simulink library "hal"  (Simulink 8.2)
settings: Solver=ode45  SolverMode=SingleTasking  StartTime=0.0  StopTime=10.0  RelTol=1e-3
PostLoadFcn:
  | , if any(exist('dsrtsu_mdlpostloadfcn', 'file') == [2, 3, 6]), try dsrtsu_mdlpostloadfcn('Execute', bdroot); catch fprintf('Error in PostLoadFcn (dsrtsu_mdlpostloadfcn) for model "%s":\n %s\n', bdroot, lasterr); end, end,
values from neighbouring files (symbols this model uses):
  INVALID_ABS1_TIMEOUT = single(0.03)    [hal_def.m]
  INVALID_ABS2_TIMEOUT = single(0.03)    [hal_def.m]
  INVALID_ABS3_TIMEOUT = single(0.03)    [hal_def.m]
  INVALID_ABS4_TIMEOUT = single(0.03)    [hal_def.m]
  INVALID_AC1_TIMEOUT = single(0.3)    [hal_def.m]
  INVALID_BCM1_TIMEOUT = single(0.6)    [hal_def.m]
  INVALID_BCM2_TIMEOUT = single(0.06)    [hal_def.m]
  INVALID_BOOSTER_VAC = uint32(255)    [hal_def.m]
  INVALID_CUR_VEHDECE = uint32(255)    [hal_def.m]
  INVALID_CURBRAKEDECE_REQ = uint32(255)    [hal_def.m]
  INVALID_CURSTEERANG_REQ = uint32(65535)    [hal_def.m]
  INVALID_CURSTEERTQ_REQ = uint32(255)    [hal_def.m]
  INVALID_ECM1_TIMEOUT = single(0.03)    [hal_def.m]
  INVALID_ECM2_TIMEOUT = single(0.03)    [hal_def.m]
  INVALID_ECM3_TIMEOUT = single(0.03)    [hal_def.m]
  INVALID_ECM9_TIMEOUT = single(0.03)    [hal_def.m]
  INVALID_ENG_TORQUE_FRICTIONAL = uint32(255)    [hal_def.m]
  INVALID_ENG_TORQUE_INDICATED = uint32(255)    [hal_def.m]
  INVALID_ENG_TORQUE_INDICATEDCOR = uint32(255)    [hal_def.m]
  INVALID_ENG_TQ_MAX = uint32(65535)    [hal_def.m]
  INVALID_ENG_TQ_MIN = uint32(65535)    [hal_def.m]
  INVALID_EPAS2_TIMEOUT = single(0.03)    [hal_def.m]
  INVALID_EPAS3_TIMEOUT = single(0.03)    [hal_def.m]
  INVALID_EPB1_TIMEOUT = single(0.12)    [hal_def.m]
  INVALID_EPS_BATTVOLT = uint32(251)    [hal_def.m]
  INVALID_ESC_BATTVOLT = uint32(251)    [hal_def.m]
  INVALID_GRADE = uint32(255)    [hal_def.m]
  INVALID_HCU3_TIMEOUT = single(0.03)    [hal_def.m]
  INVALID_HCU4_TIMEOUT = single(0.03)    [hal_def.m]
  INVALID_HMI1_TIMEOUT = single(0.03)    [hal_def.m]
  INVALID_HMI2_TIMEOUT = single(0.03)    [hal_def.m]
  INVALID_LAT_ACC = uint32(255)    [hal_def.m]
  INVALID_LONG_ACC = uint32(255)    [hal_def.m]
  INVALID_MC_PRESSURE = uint32(2047)    [hal_def.m]
  INVALID_METER1_TIMEOUT = single(0.3)    [hal_def.m]
  INVALID_METER3_TIMEOUT = single(0.3)    [hal_def.m]
  INVALID_METER_VEHSPD = uint32(2048)    [hal_def.m]
  INVALID_ODO_METER = uint32(1000000)    [hal_def.m]
  INVALID_OUTSIDE_TEMP = uint32(96)    [hal_def.m]
  INVALID_PARKBRAKEBIND_STAT = uint32(3)    [hal_def.m]
  INVALID_SAS1_TIMEOUT = single(0.03)    [hal_def.m]
  INVALID_SAS_ANGLE = uint32(65535)    [hal_def.m]
  INVALID_SHIFTER_POSN = uint32(6)    [hal_def.m]
  INVALID_TCM1_TIMEOUT = single(0.03)    [hal_def.m]
  INVALID_TCM2_TIMEOUT = single(0.03)    [hal_def.m]
  INVALID_VCU1_TIMEOUT = single(0.03)    [hal_def.m]
  INVALID_VCU2_TIMEOUT = single(0.03)    [hal_def.m]
  INVALID_VEH_CRASH = uint32(15)    [hal_def.m]
  INVALID_VEH_SPD = uint32(2048)    [hal_def.m]
  INVALID_WHEEL_SPD = uint32(16377)    [hal_def.m]
  INVALID_YAW_RATE = uint32(2001)    [hal_def.m]
undefined symbols (not defined in the file or in its folder): C_TASK_5MS_S, FALSE, INVALID_CURPTTORQ_REQ, KHAL_MssgIdObj1_num, KHAL_MssgIdObj2_num, KHAL_MssgIdObjStatus_num, TRUE
libraries: simulink x92
(part 8 of 8)

== system hal/dHAL_IN/dHAL_IN_ABS/BO_864_ABS2_8_ABS/IcM ==
  LowByte : Inport
  HighByte : Inport  Port=2
  Bitwise Operator : simulink/Logic and Bit Operations/Bitwise Operator  logicop=OR  UseBitMask=off  NumInputPorts=2  BitMask=bin2dec('11011001')  BitMaskRealWorld=Stored Integer
  Cast1 : DataTypeConversion  OutDataTypeStr=uint16  RndMeth=Zero
  Cast45 : DataTypeConversion  OutDataTypeStr=uint16  RndMeth=Zero
  Shift Arithmetic : ArithShift  BitShiftNumber=-4
  Shift Arithmetic1 : ArithShift  BitShiftNumber=4
  HighLowByte : Outport
  wires:
  Shift Arithmetic1/1 -> Bitwise Operator/2
  LowByte/1 -> Cast1/1
  Cast1/1 -> Shift Arithmetic1/1
  Cast45/1 -> Shift Arithmetic/1
  HighByte/1 -> Cast45/1
  Bitwise Operator/1 -> HighLowByte/1
  Shift Arithmetic/1 -> Bitwise Operator/1

== system hal/dHAL_IN/dHAL_IN_ABS/BO__880_ABS3__8_ABS/IcM ==
  LowByte : Inport
  HighByte : Inport  Port=2
  Bitwise Operator : simulink/Logic and Bit Operations/Bitwise Operator  logicop=OR  UseBitMask=off  NumInputPorts=2  BitMask=bin2dec('11011001')  BitMaskRealWorld=Stored Integer
  Cast1 : DataTypeConversion  OutDataTypeStr=uint16  RndMeth=Zero
  Cast45 : DataTypeConversion  OutDataTypeStr=uint16  RndMeth=Zero
  Shift Arithmetic : ArithShift  BitShiftNumber=-7
  Shift Arithmetic1 : ArithShift  BitShiftNumber=1
  HighLowByte : Outport
  wires:
  Shift Arithmetic1/1 -> Bitwise Operator/2
  LowByte/1 -> Cast1/1
  Cast1/1 -> Shift Arithmetic1/1
  Cast45/1 -> Shift Arithmetic/1
  HighByte/1 -> Cast45/1
  Bitwise Operator/1 -> HighLowByte/1
  Shift Arithmetic/1 -> Bitwise Operator/1

== system hal/dHAL_IN/dHAL_IN_ABS/BO__880_ABS3__8_ABS/IcM1 ==
  LowByte : Inport
  HighByte : Inport  Port=2
  Bitwise Operator : simulink/Logic and Bit Operations/Bitwise Operator  logicop=OR  UseBitMask=off  NumInputPorts=2  BitMask=bin2dec('11011001')  BitMaskRealWorld=Stored Integer
  Cast1 : DataTypeConversion  OutDataTypeStr=uint16  RndMeth=Zero
  Cast45 : DataTypeConversion  OutDataTypeStr=uint16  RndMeth=Zero
  Shift Arithmetic : ArithShift  BitShiftNumber=-7
  Shift Arithmetic1 : ArithShift  BitShiftNumber=1
  HighLowByte : Outport
  wires:
  Shift Arithmetic/1 -> Bitwise Operator/1
  Bitwise Operator/1 -> HighLowByte/1
  HighByte/1 -> Cast45/1
  Cast45/1 -> Shift Arithmetic/1
  Cast1/1 -> Shift Arithmetic1/1
  LowByte/1 -> Cast1/1
  Shift Arithmetic1/1 -> Bitwise Operator/2

== system hal/dHAL_IN/dHAL_IN_ABS/BO__880_ABS3__8_ABS/IcM2 ==
  LowByte : Inport
  HighByte : Inport  Port=2
  Bitwise Operator : simulink/Logic and Bit Operations/Bitwise Operator  logicop=OR  UseBitMask=off  NumInputPorts=2  BitMask=bin2dec('11011001')  BitMaskRealWorld=Stored Integer
  Cast1 : DataTypeConversion  OutDataTypeStr=uint16  RndMeth=Zero
  Cast45 : DataTypeConversion  OutDataTypeStr=uint16  RndMeth=Zero
  Shift Arithmetic : ArithShift  BitShiftNumber=-7
  Shift Arithmetic1 : ArithShift  BitShiftNumber=1
  HighLowByte : Outport
  wires:
  Shift Arithmetic1/1 -> Bitwise Operator/2
  LowByte/1 -> Cast1/1
  Cast1/1 -> Shift Arithmetic1/1
  Cast45/1 -> Shift Arithmetic/1
  HighByte/1 -> Cast45/1
  Bitwise Operator/1 -> HighLowByte/1
  Shift Arithmetic/1 -> Bitwise Operator/1

== system hal/dHAL_IN/dHAL_IN_ABS/BO__880_ABS3__8_ABS/IcM3 ==
  LowByte : Inport
  HighByte : Inport  Port=2
  Bitwise Operator : simulink/Logic and Bit Operations/Bitwise Operator  logicop=OR  UseBitMask=off  NumInputPorts=2  BitMask=bin2dec('11011001')  BitMaskRealWorld=Stored Integer
  Cast1 : DataTypeConversion  OutDataTypeStr=uint16  RndMeth=Zero
  Cast45 : DataTypeConversion  OutDataTypeStr=uint16  RndMeth=Zero
  Shift Arithmetic : ArithShift  BitShiftNumber=-7
  Shift Arithmetic1 : ArithShift  BitShiftNumber=1
  HighLowByte : Outport
  wires:
  Shift Arithmetic/1 -> Bitwise Operator/1
  Bitwise Operator/1 -> HighLowByte/1
  HighByte/1 -> Cast45/1
  Cast45/1 -> Shift Arithmetic/1
  Cast1/1 -> Shift Arithmetic1/1
  LowByte/1 -> Cast1/1
  Shift Arithmetic1/1 -> Bitwise Operator/2

== system hal/dHAL_IN/dHAL_IN_ABS/BO__896_ABS4__8_ABS/IcM ==
  LowByte : Inport
  HighByte : Inport  Port=2
  Bitwise Operator : simulink/Logic and Bit Operations/Bitwise Operator  logicop=OR  UseBitMask=off  NumInputPorts=2  BitMask=bin2dec('11011001')  BitMaskRealWorld=Stored Integer
  Cast1 : DataTypeConversion  OutDataTypeStr=uint16  RndMeth=Zero
  Cast45 : DataTypeConversion  OutDataTypeStr=uint16  RndMeth=Zero
  Shift Arithmetic : ArithShift  BitShiftNumber=-8
  HighLowByte : Outport
  wires:
  Shift Arithmetic/1 -> Bitwise Operator/1
  Bitwise Operator/1 -> HighLowByte/1
  HighByte/1 -> Cast45/1
  Cast45/1 -> Shift Arithmetic/1
  Cast1/1 -> Bitwise Operator/2
  LowByte/1 -> Cast1/1

== system hal/dHAL_IN/dHAL_IN_ABS/BO__896_ABS4__8_ABS/IcM1 ==
  LowByte : Inport
  HighByte : Inport  Port=2
  Bitwise Operator : simulink/Logic and Bit Operations/Bitwise Operator  logicop=OR  UseBitMask=off  NumInputPorts=2  BitMask=bin2dec('11011001')  BitMaskRealWorld=Stored Integer
  Cast1 : DataTypeConversion  OutDataTypeStr=uint16  RndMeth=Zero
  Cast45 : DataTypeConversion  OutDataTypeStr=uint16  RndMeth=Zero
  Shift Arithmetic : ArithShift  BitShiftNumber=-3
  HighLowByte : Outport
  wires:
  LowByte/1 -> Cast1/1
  Cast1/1 -> Bitwise Operator/2
  Cast45/1 -> Shift Arithmetic/1
  HighByte/1 -> Cast45/1
  Bitwise Operator/1 -> HighLowByte/1
  Shift Arithmetic/1 -> Bitwise Operator/1

== system hal/dHAL_IN/dHAL_IN_ECM/BO_875_ECM9_8_ECM/IcM ==
  LowByte : Inport
  HighByte : Inport  Port=2
  Bitwise Operator : simulink/Logic and Bit Operations/Bitwise Operator  logicop=OR  UseBitMask=off  NumInputPorts=2  BitMask=bin2dec('11011001')  BitMaskRealWorld=Stored Integer
  Cast1 : DataTypeConversion  OutDataTypeStr=uint16  RndMeth=Zero
  Cast45 : DataTypeConversion  OutDataTypeStr=uint16  RndMeth=Zero
  Shift Arithmetic : ArithShift  BitShiftNumber=-8
  HighLowByte : Outport
  wires:
  Shift Arithmetic/1 -> Bitwise Operator/1
  Bitwise Operator/1 -> HighLowByte/1
  HighByte/1 -> Cast45/1
  Cast45/1 -> Shift Arithmetic/1
  Cast1/1 -> Bitwise Operator/2
  LowByte/1 -> Cast1/1

== system hal/dHAL_IN/dHAL_IN_ECM/BO_875_ECM9_8_ECM/IcM1 ==
  LowByte : Inport
  HighByte : Inport  Port=2
  Bitwise Operator : simulink/Logic and Bit Operations/Bitwise Operator  logicop=OR  UseBitMask=off  NumInputPorts=2  BitMask=bin2dec('11011001')  BitMaskRealWorld=Stored Integer
  Cast1 : DataTypeConversion  OutDataTypeStr=uint16  RndMeth=Zero
  Cast45 : DataTypeConversion  OutDataTypeStr=uint16  RndMeth=Zero
  Shift Arithmetic : ArithShift  BitShiftNumber=-8
  HighLowByte : Outport
  wires:
  LowByte/1 -> Cast1/1
  Cast1/1 -> Bitwise Operator/2
  Cast45/1 -> Shift Arithmetic/1
  HighByte/1 -> Cast45/1
  Bitwise Operator/1 -> HighLowByte/1
  Shift Arithmetic/1 -> Bitwise Operator/1

== system hal/dHAL_IN/dHAL_IN_EPAS/BO__1365_EPAS3__8_EPAS/ChecksumCalculation ==
  EPAS3_LifeCount : Inport
  CAN1_Rx : Inport  Port=2
  Bitwise Operator1 : simulink/Logic and Bit Operations/Bitwise Operator  logicop=XOR  UseBitMask=off  NumInputPorts=4  BitMask=bin2dec('11011001')  BitMaskRealWorld=Stored Integer
  Bitwise Operator2 : simulink/Logic and Bit Operations/Bitwise Operator  logicop=XOR  UseBitMask=off  NumInputPorts=3  BitMask=bin2dec('11011001')  BitMaskRealWorld=Stored Integer
  Bus Selector : BusSelector  OutputSignals=EPAS3.RAW_Byte_1,EPAS3.RAW_Byte_2,EPAS3.RAW_Byte_3,EPAS3.RAW_Byte_4
  Data Type Conversion{1,3,6..9} (6 alike) : DataTypeConversion  OutDataTypeStr=uint8
  Extract Bits5 : simulink/Logic and Bit Operations/Extract Bits  bitsToExtract=Lower half  numBits=8  bitIdxRange=[0 7]  outScalingMode=Preserve fixed-point scaling
  Extract Bits6 : simulink/Logic and Bit Operations/Extract Bits  bitsToExtract=Upper half  numBits=8  bitIdxRange=[0 7]  outScalingMode=Preserve fixed-point scaling
  Shift Arithmetic2 : ArithShift  BitShiftNumber=4
  Message_Checksum : Outport
  wires:
  Bus Selector/2 -> Data Type Conversion3/1  "<RAW_Byte_2>"
  Extract Bits6/1 -> Data Type Conversion7/1
  Extract Bits5/1 -> Data Type Conversion8/1
  Data Type Conversion7/1 -> Shift Arithmetic2/1
  Bus Selector/3 -> Data Type Conversion6/1  "<RAW_Byte_3>"
  Bus Selector/4 -> Data Type Conversion9/1  "<RAW_Byte_4>"
  Bus Selector/1 -> Data Type Conversion1/1  "<RAW_Byte_1>"
  Data Type Conversion1/1 -> Bitwise Operator1/1
  Data Type Conversion3/1 -> Bitwise Operator1/2
  Data Type Conversion6/1 -> Bitwise Operator1/3
  Data Type Conversion9/1 -> Bitwise Operator1/4
  Bitwise Operator1/1 -> Extract Bits6/1, Extract Bits5/1
  Shift Arithmetic2/1 -> Bitwise Operator2/1
  Data Type Conversion8/1 -> Bitwise Operator2/2
  EPAS3_LifeCount/1 -> Bitwise Operator2/3
  Bitwise Operator2/1 -> Message_Checksum/1
  CAN1_Rx/1 -> [CAN1_Rx]
  [CAN1_Rx] -> Bus Selector/1

== system hal/dHAL_IN/dHAL_IN_EPAS/BO__1365_EPAS3__8_EPAS/IcM ==
  LowByte : Inport
  HighByte : Inport  Port=2
  Bitwise Operator : simulink/Logic and Bit Operations/Bitwise Operator  logicop=OR  UseBitMask=off  NumInputPorts=2  BitMask=bin2dec('11011001')  BitMaskRealWorld=Stored Integer
  Cast1 : DataTypeConversion  OutDataTypeStr=uint16  RndMeth=Zero
  Cast45 : DataTypeConversion  OutDataTypeStr=uint16  RndMeth=Zero
  Shift Arithmetic : ArithShift  BitShiftNumber=-8
  HighLowByte : Outport
  wires:
  LowByte/1 -> Cast1/1
  Cast1/1 -> Bitwise Operator/2
  Cast45/1 -> Shift Arithmetic/1
  HighByte/1 -> Cast45/1
  Bitwise Operator/1 -> HighLowByte/1
  Shift Arithmetic/1 -> Bitwise Operator/1

== system hal/dHAL_IN/dHAL_IN_EPAS/BO__922_SAS1__8_EPAS/ChecksumCalculation ==
  SAS_MsgCount : Inport
  CAN1_Rx : Inport  Port=2
  Bitwise Operator1 : simulink/Logic and Bit Operations/Bitwise Operator  logicop=XOR  UseBitMask=off  NumInputPorts=4  BitMask=bin2dec('11011001')  BitMaskRealWorld=Stored Integer
  Bitwise Operator2 : simulink/Logic and Bit Operations/Bitwise Operator  logicop=XOR  UseBitMask=off  NumInputPorts=3  BitMask=bin2dec('11011001')  BitMaskRealWorld=Stored Integer
  Bus Selector : BusSelector  OutputSignals=SAS1.RAW_Byte_1,SAS1.RAW_Byte_2,SAS1.RAW_Byte_3,SAS1.RAW_Byte_4
  Data Type Conversion{1..3,6..9} (7 alike) : DataTypeConversion  OutDataTypeStr=uint8
  Extract Bits5 : simulink/Logic and Bit Operations/Extract Bits  bitsToExtract=Lower half  numBits=8  bitIdxRange=[0 7]  outScalingMode=Preserve fixed-point scaling
  Extract Bits6 : simulink/Logic and Bit Operations/Extract Bits  bitsToExtract=Upper half  numBits=8  bitIdxRange=[0 7]  outScalingMode=Preserve fixed-point scaling
  Shift Arithmetic2 : ArithShift  BitShiftNumber=4
  Message_Checksum : Outport
  wires:
  Data Type Conversion2/1 -> Bitwise Operator2/3
  CAN1_Rx/1 -> Bus Selector/1
  Bitwise Operator2/1 -> Message_Checksum/1
  SAS_MsgCount/1 -> Data Type Conversion2/1
  Data Type Conversion8/1 -> Bitwise Operator2/2
  Shift Arithmetic2/1 -> Bitwise Operator2/1
  Bitwise Operator1/1 -> Extract Bits5/1, Extract Bits6/1
  Data Type Conversion9/1 -> Bitwise Operator1/4
  Data Type Conversion6/1 -> Bitwise Operator1/3
  Data Type Conversion3/1 -> Bitwise Operator1/2
  Data Type Conversion1/1 -> Bitwise Operator1/1
  Bus Selector/1 -> Data Type Conversion1/1  "<RAW_Byte_1>"
  Bus Selector/4 -> Data Type Conversion9/1  "<RAW_Byte_4>"
  Bus Selector/3 -> Data Type Conversion6/1  "<RAW_Byte_3>"
  Data Type Conversion7/1 -> Shift Arithmetic2/1
  Extract Bits5/1 -> Data Type Conversion8/1
  Extract Bits6/1 -> Data Type Conversion7/1
  Bus Selector/2 -> Data Type Conversion3/1  "<RAW_Byte_2>"

== system hal/dHAL_IN/dHAL_IN_EPAS/BO__922_SAS1__8_EPAS/IcM ==
  LowByte : Inport
  HighByte : Inport  Port=2
  Bitwise Operator : simulink/Logic and Bit Operations/Bitwise Operator  logicop=OR  UseBitMask=off  NumInputPorts=2  BitMask=bin2dec('11011001')  BitMaskRealWorld=Stored Integer
  Cast1 : DataTypeConversion  OutDataTypeStr=uint16  RndMeth=Zero
  Cast45 : DataTypeConversion  OutDataTypeStr=uint16  RndMeth=Zero
  Shift Arithmetic : ArithShift  BitShiftNumber=-8
  HighLowByte : Outport
  wires:
  Shift Arithmetic/1 -> Bitwise Operator/1
  Bitwise Operator/1 -> HighLowByte/1
  HighByte/1 -> Cast45/1
  Cast45/1 -> Shift Arithmetic/1
  Cast1/1 -> Bitwise Operator/2
  LowByte/1 -> Cast1/1

== system hal/dHAL_IN/dHAL_IN_EPAS/BO__926_EPAS2__8_EPAS/ChecksumCalculation ==
  SAS_MsgCount : Inport
  CAN1_Rx : Inport  Port=2
  Bitwise Operator1 : simulink/Logic and Bit Operations/Bitwise Operator  logicop=XOR  UseBitMask=off  NumInputPorts=4  BitMask=bin2dec('11011001')  BitMaskRealWorld=Stored Integer
  Bitwise Operator2 : simulink/Logic and Bit Operations/Bitwise Operator  logicop=XOR  UseBitMask=off  NumInputPorts=3  BitMask=bin2dec('11011001')  BitMaskRealWorld=Stored Integer
  Bus Selector : BusSelector  OutputSignals=EPAS2.RAW_Byte_1,EPAS2.RAW_Byte_2,EPAS2.RAW_Byte_3,EPAS2.RAW_Byte_4
  Data Type Conversion{1,3,6..9} (6 alike) : DataTypeConversion  OutDataTypeStr=uint8
  Extract Bits5 : simulink/Logic and Bit Operations/Extract Bits  bitsToExtract=Lower half  numBits=8  bitIdxRange=[0 7]  outScalingMode=Preserve fixed-point scaling
  Extract Bits6 : simulink/Logic and Bit Operations/Extract Bits  bitsToExtract=Upper half  numBits=8  bitIdxRange=[0 7]  outScalingMode=Preserve fixed-point scaling
  Shift Arithmetic2 : ArithShift  BitShiftNumber=4
  Message_Checksum : Outport
  wires:
  [CAN1_Rx] -> Bus Selector/1
  CAN1_Rx/1 -> [CAN1_Rx]
  Bitwise Operator2/1 -> Message_Checksum/1
  SAS_MsgCount/1 -> Bitwise Operator2/3
  Data Type Conversion8/1 -> Bitwise Operator2/2
  Shift Arithmetic2/1 -> Bitwise Operator2/1
  Bitwise Operator1/1 -> Extract Bits5/1, Extract Bits6/1
  Data Type Conversion9/1 -> Bitwise Operator1/4
  Data Type Conversion6/1 -> Bitwise Operator1/3
  Data Type Conversion3/1 -> Bitwise Operator1/2
  Data Type Conversion1/1 -> Bitwise Operator1/1
  Bus Selector/1 -> Data Type Conversion1/1  "<RAW_Byte_1>"
  Bus Selector/4 -> Data Type Conversion9/1  "<RAW_Byte_4>"
  Bus Selector/3 -> Data Type Conversion6/1  "<RAW_Byte_3>"
  Data Type Conversion7/1 -> Shift Arithmetic2/1
  Extract Bits5/1 -> Data Type Conversion8/1
  Extract Bits6/1 -> Data Type Conversion7/1
  Bus Selector/2 -> Data Type Conversion3/1  "<RAW_Byte_2>"

== system hal/dHAL_IN/dHAL_IN_EPAS/BO__926_EPAS2__8_EPAS/IcM ==
  LowByte : Inport
  HighByte : Inport  Port=2
  Bitwise Operator : simulink/Logic and Bit Operations/Bitwise Operator  logicop=OR  UseBitMask=off  NumInputPorts=2  BitMask=bin2dec('11011001')  BitMaskRealWorld=Stored Integer
  Cast1 : DataTypeConversion  OutDataTypeStr=uint16  RndMeth=Zero
  Cast45 : DataTypeConversion  OutDataTypeStr=uint16  RndMeth=Zero
  Shift Arithmetic : ArithShift  BitShiftNumber=-8
  HighLowByte : Outport
  wires:
  Shift Arithmetic/1 -> Bitwise Operator/1
  Bitwise Operator/1 -> HighLowByte/1
  HighByte/1 -> Cast45/1
  Cast45/1 -> Shift Arithmetic/1
  Cast1/1 -> Bitwise Operator/2
  LowByte/1 -> Cast1/1

== system hal/dHAL_IN/dHAL_IN_METER/BO__1306_Meter3__8_Meter/IcM ==
  LowByte : Inport
  HighByte : Inport  Port=2
  Bitwise Operator : simulink/Logic and Bit Operations/Bitwise Operator  logicop=OR  UseBitMask=off  NumInputPorts=2  BitMask=bin2dec('11011001')  BitMaskRealWorld=Stored Integer
  Cast1 : DataTypeConversion  OutDataTypeStr=uint16  RndMeth=Zero
  Cast45 : DataTypeConversion  OutDataTypeStr=uint16  RndMeth=Zero
  Shift Arithmetic : ArithShift  BitShiftNumber=-4
  Shift Arithmetic1 : ArithShift  BitShiftNumber=4
  HighLowByte : Outport
  wires:
  Shift Arithmetic1/1 -> Bitwise Operator/2
  LowByte/1 -> Cast1/1
  Cast1/1 -> Shift Arithmetic1/1
  Cast45/1 -> Shift Arithmetic/1
  HighByte/1 -> Cast45/1
  Bitwise Operator/1 -> HighLowByte/1
  Shift Arithmetic/1 -> Bitwise Operator/1

== system hal/dHAL_IN/HAL_IN_RadObjDecoder/RObjectPackFrame/RObjects_Decoder_v2/CheckIDs ==
  Status : Inport
  ID : Inport  Port=2
  R_Objects_in : Inport  Port=3  OutDataTypeStr=Bus: R_Objects
  CAN_RAW_Deco : Stateflow chart  TreatAsAtomicUnit=on
  R_Objects_out : Outport  OutDataTypeStr=Bus: R_Objects
  ParseFrame : Outport  Port=2
  wires:
  Status/1 -> CAN_RAW_Deco/1(Status)
  ID/1 -> CAN_RAW_Deco/2(ID)
  CAN_RAW_Deco/2(ParseFrames()) -> ParseFrame/1
  R_Objects_in/1 -> CAN_RAW_Deco/3(R_Objects_in)
  CAN_RAW_Deco/1(R_Objects_out) -> R_Objects_out/1

== system hal/dHAL_IN/HAL_IN_RadObjDecoder/RObjectPackFrame/RObjects_Decoder_v2/ParseFrames ==
  R_Objects_in : Inport  OutDataTypeStr=Bus: R_Objects
  Byte1 : Inport  Port=2
  Byte2 : Inport  Port=3
  Byte3 : Inport  Port=4
  Byte4 : Inport  Port=5
  Byte5 : Inport  Port=6
  Byte6 : Inport  Port=7
  Byte7 : Inport  Port=8
  Byte8 : Inport  Port=9
  Trigger : TriggerPort  TriggerType=function-call  PortDimensions=1
  MATLAB Function : MATLAB Function  TreatAsAtomicUnit=on
  R_Objects_out : Outport  OutDataTypeStr=Bus: R_Objects
  wires:
  Byte7/1 -> MATLAB Function/8(Byte7)
  Byte1/1 -> MATLAB Function/2(Byte1)
  Byte5/1 -> MATLAB Function/6(Byte5)
  Byte6/1 -> MATLAB Function/7(Byte6)
  Byte8/1 -> MATLAB Function/9(Byte8)
  Byte4/1 -> MATLAB Function/5(Byte4)
  Byte3/1 -> MATLAB Function/4(Byte3)
  Byte2/1 -> MATLAB Function/3(Byte2)
  R_Objects_in/1 -> MATLAB Function/1(R_Objects_in)
  MATLAB Function/1(R_Objects_out) -> R_Objects_out/1

== matlab function dHAL_IN/HAL_IN_RadObjDecoder/RObj_Parser/RObj_FramesParser ==
  data: Frames1 input uint8; Obj_RolCount output uint8; Obj_ID output uint8; Obj_LongDispl output single; Obj_VrelLong output single; Obj_AccelLong output single; Obj_LatDispl output single; Obj_DynProp output uint8; Obj_ProbOfExist output uint8; Obj_MeasStat output uint8; Obj_Width output uint8; Obj_Length output uint8; Frames2 input uint8; Obj_RCSValue output single; Obj_LatSpeed output single; Obj_ObstacleProb output uint8
function [Obj_RolCount,Obj_ID, Obj_LongDispl, Obj_VrelLong, Obj_AccelLong, Obj_LatDispl, Obj_DynProp, Obj_ProbOfExist, Obj_MeasStat, Obj_Width, Obj_Length, Obj_RCSValue, Obj_LatSpeed, Obj_ObstacleProb] = fcn(Frames1, Frames2)

NofObjects = uint8(40);
Obj_RolCount = uint8(zeros(1,40));
Obj_ID = uint8(zeros(1,40));
Obj_LongDispl = single(zeros(1,40));
Obj_VrelLong = single(zeros(1,40));
Obj_AccelLong = single(zeros(1,40));
Obj_LatDispl = single(zeros(1,40));
Obj_ProbOfExist = uint8(zeros(1,40));
Obj_DynProp = uint8(zeros(1,40));
Obj_MeasStat = uint8(zeros(1,40));
Obj_RCSValue = single(zeros(1,40));
Obj_LatSpeed = single(zeros(1,40));
Obj_ObstacleProb = uint8(zeros(1,40));
Obj_Length = uint8(zeros(1,40));
Obj_Width = uint8(zeros(1,40));

%%%%%%%%%%%%%%%%%%%%%%%%%%%%%%%
%%%%%%%%%%%% FRAMES1 %%%%%%%%%%
%%%%%%%%%%%%%%%%%%%%%%%%%%%%%%%

Obj_RollCount_Mask = uint8(bin2dec ('00000011'));
Obj_ID_Mask = uint8(bin2dec('11111100'));
Obj_LongDispl_Mask = uint8(bin2dec('11100000'));
Obj_VrelLong_b1_Mask = uint8(bin2dec('00011111'));
Obj_VrelLong_b2_Mask = uint8(bin2dec('11111110'));
Obj_AccelLong_b1_Mask = uint8(bin2dec('000000001'));
Obj_LatDispl_b2_Mask = uint8(bin2dec('11000000'));
Obj_DynProp_b1_Mask = uint8(bin2dec('00111000'));
Obj_ProbOfExist_b1_Mask = uint8(bin2dec('00000111'));
Obj_MeasStat_b1_Mask = uint8(bin2dec('11000000'));
Obj_Width_b1_Mask = uint8(bin2dec('00111000'));
Obj_Length_b1_Mask = uint8(bin2dec('00000111'));

for Obj_Count = 1:NofObjects

Obj_RolCount(1,Obj_Count) = bitand(uint8(Frames1(1,Obj_Count)),Obj_RollCount_Mask);     
Obj_ID(1,Obj_Count) = bitshift(bitand(Frames1(1,Obj_Count),Obj_ID_Mask),-2);

Obj_LongDispl_2byte = uint16(bitshift(bitand(Frames1(3,Obj_Count),Obj_LongDispl_Mask),-5));
Obj_LongDispl_u16 = uint16(bitshift(uint16(Frames1(2,Obj_Count)),3));
Obj_LongDispl_u16 = uint16(bitor(Obj_LongDispl_u16,Obj_LongDispl_2byte));
Obj_LongDispl(1,Obj_Count) = single(single(Obj_LongDispl_u16)*0.1);

Obj_VrelLong_byte1 = uint16(bitshift(bitand(uint16(Frames1(3,Obj_Count)),uint16(Obj_VrelLong_b1_Mask)),7));
Obj_VrelLong_byte2 = uint16(bitshift(bitand(Frames1(4,Obj_Count),Obj_VrelLong_b2_Mask),-1));
Obj_VrelLong_u16 = uint16(bitor(Obj_VrelLong_byte1,Obj_VrelLong_byte2));
Obj_VrelLong(1,Obj_Count) = single(single(Obj_VrelLong_u16)*0.0625);
Obj_VrelLong(1,Obj_Count) = Obj_VrelLong(1,Obj_Count) - 128;

Obj_AccelLong_byte1 = uint16(bitand(uint16(Frames1(4,Obj_Count)),uint16(Obj_AccelLong_b1_Mask)));
Obj_AccelLong_u16 = uint16(bitor(Obj_AccelLong_byte1,uint16(Frames1(5,Obj_Count))));
Obj_AccelLong(1,Obj_Count) = single(single(Obj_AccelLong_u16)*0.0625);
Obj_AccelLong(1,Obj_Count) = Obj_AccelLong(1,Obj_Count) - 16;


Obj_LatDispl_byte2 = uint16(bitand(uint16(Frames1(7,Obj_Count)),uint16(Obj_LatDispl_b2_Mask)));
Obj_LatDispl_byte2 = bitshift(Obj_LatDispl_byte2,-6);
Obj_LatDispl_byte1 = uint16(bitshift(uint16(Frames1(6,Obj_Count)),2));
Obj_LatDispl_u16 = uint16(bitor(Obj_LatDispl_byte1,Obj_LatDispl_byte2));
Obj_LatDispl(1,Obj_Count) = single(single(Obj_LatDispl_u16) * 0.1);
Obj_LatDispl(1,Obj_Count) = Obj_LatDispl(1,Obj_Count) - 52;

Obj_ProbOfExist(1,Obj_Count) = uint8(bitand(Frames1(7,Obj_Count),Obj_ProbOfExist_b1_Mask));

Obj_DynProp(1,Obj_Count) = uint8(bitand(Frames1(7,Obj_Count),Obj_DynProp_b1_Mask));
Obj_DynProp(1,Obj_Count) = uint8(bitshift(Obj_DynProp(1,Obj_Count),-3));

Obj_Length(1,Obj_Count) = uint8(bitand(Frames1(8,Obj_Count),Obj_Length_b1_Mask));

Obj_Width(1,Obj_Count) = uint8(bitand(Frames1(8,Obj_Count),Obj_Width_b1_Mask));
Obj_Width(1,Obj_Count) = uint8(bitshift(Obj_Width(1,Obj_Count),-3));

Obj_MeasStat(1,Obj_Count) = uint8(bitand(Frames1(8,Obj_Count),Obj_MeasStat_b1_Mask));
Obj_MeasStat(1,Obj_Count) = uint8(bitshift(Obj_MeasStat(1,Obj_Count),-6));

%%%%%%%%%%%%%%%%%%%%%%%%%%%%%%%
%%%%%%%%%%%% FRAMES2 %%%%%%%%%%
%%%%%%%%%%%%%%%%%%%%%%%%%%%%%%%

Obj_ObstacleProb_b1_Mask = uint8(bin2dec('01111111'));

Obj_RCSValue(1,Obj_Count) = (single(Frames2(1,Obj_Count))*0.5)-64;
Obj_LatSpeed(1,Obj_Count) = (single(Frames2(2,Obj_Count))*0.25)-32;
Obj_ObstacleProb(1,Obj_Count) = uint8(bitand(Frames2(3,Obj_Count),Obj_ObstacleProb_b1_Mask));

end

end

== matlab function dHAL_IN/HAL_IN_RadObjDecoder/RObj_Parser/RObj_StatusParser ==
  data: Status_Frame input uint8 size=8; N_of_Objects output uint8; MeasCounter output uint16; SensorRxInvalid output uint8; SensorSupplyVoltage output uint8; SensorDefective output uint8; SensorMisaligned output uint8; SensorSwitchedOff output uint8; SensorExternalDisturbed output uint8; SensorOutputReduced output uint8; LatDistToborderLeft output single; LatDistToborderRight output single
function [N_of_Objects,MeasCounter, SensorRxInvalid, SensorSupplyVoltage, SensorDefective, SensorMisaligned, SensorSwitchedOff, SensorExternalDisturbed, SensorOutputReduced, LatDistToborderLeft, LatDistToborderRight] = fcn(Status_Frame)


N_of_Objects = uint8(Status_Frame(1,1));

MeasCounter = typecast([Status_Frame(2,1) Status_Frame(3,1)],'uint16');   

SensorRxInvalid = bitget(Status_Frame(4,1),7);
SensorSupplyVoltage = bitget(Status_Frame(4,1),6);
SensorDefective = bitget(Status_Frame(4,1),5);
SensorMisaligned = bitget(Status_Frame(4,1),4);
SensorSwitchedOff = bitget(Status_Frame(4,1),3);
SensorExternalDisturbed = bitget(Status_Frame(4,1),2);
SensorOutputReduced = bitget(Status_Frame(4,1),1);
LatDistToborderLeft = single(single(Status_Frame(6,1))*0.1);
LatDistToborderRight = single(single(Status_Frame(7,1))*0.1);



end

== stateflow chart dHAL_IN/HAL_IN_RadObjDecoder/RObjectPackFrame/RObjects_Decoder_v2/CheckIDs/CAN_RAW_Deco ==
  (default) -> (junction 51)
  (junction 51) -> (junction 53) : {
      | R_Objects_out = R_Objects_in;
      | }
  (junction 54) -> (junction 52) [order 1] : [ID == KHAL_MssgIdObjStatus_num]
  (junction 53) -> (junction 54) [order 1] : [Status == TRUE]
  (junction 52) -> (junction 65) : {
      | R_Objects_out.ObS_on = true;
      | R_Objects_out.ObF1_on = false;
      | R_Objects_out.ObF2_on = false;
      | }
  (junction 53) -> (junction 59) [order 2]
  (junction 54) -> (junction 55) [order 2]
  (junction 55) -> (junction 56) [order 1] : [ID == KHAL_MssgIdObj1_num]
  (junction 55) -> (junction 57) [order 2]
  (junction 56) -> (junction 64) : {
      | R_Objects_out.ObS_on = false;
      | R_Objects_out.ObF1_on = true;
      | R_Objects_out.ObF2_on = false;
      | }
  (junction 57) -> (junction 58) : [ID == KHAL_MssgIdObj2_num]
  (junction 58) -> (junction 63) : {
      | R_Objects_out.ObS_on = false;
      | R_Objects_out.ObF1_on = false;
      | R_Objects_out.ObF2_on = true;
      | }
  (junction 59) -> (junction 60) [order 1] : [Status == FALSE]
  (junction 59) -> (junction 61) [order 2]
  (junction 60) -> (junction 62) : {
      | R_Objects_out.ObS_on = false;
      | R_Objects_out.ObF1_on = false;
      | R_Objects_out.ObF2_on = false;
      | }
  (junction 62) -> (junction 61)
  (junction 63) -> (junction 62)
  (junction 64) -> (junction 63)
  (junction 65) -> (junction 64)
  (junction 61) -> (junction 66) : {
      | ParseFrames;
      | }
  (junction 66) -> (junction 67)
  data: Status input boolean; ID input uint32; KHAL_MssgIdObj1_num parameter double; KHAL_MssgIdObj2_num parameter double; KHAL_MssgIdObjStatus_num parameter double; R_Objects_in input Bus: R_Objects; R_Objects_out output Bus: R_Objects; TRUE parameter boolean; FALSE parameter boolean
  events: ParseFrames output FUNCTION_CALL_EVENT

== matlab function dHAL_IN/HAL_IN_RadObjDecoder/RObjectPackFrame/RObjects_Decoder_v2/ParseFrames/MATLAB Function ==
  data: R_Objects_in input Bus: R_Objects; Byte1 input uint8; Byte2 input uint8; Byte3 input uint8; Byte4 input uint8; Byte5 input uint8; Byte6 input uint8; Byte7 input uint8; Byte8 input uint8; R_Objects_out output Bus: R_Objects
function R_Objects_out  = fcn(R_Objects_in, Byte1, Byte2, Byte3, Byte4, Byte5, Byte6, Byte7, Byte8)


R_Objects_out = R_Objects_in;

if (R_Objects_in.ObS_on == true)

R_Objects_out.StatusFrame(1,1) =  uint8(Byte1);
R_Objects_out.StatusFrame(1,2) =  uint8(Byte2);
R_Objects_out.StatusFrame(1,3) =  uint8(Byte3);
R_Objects_out.StatusFrame(1,4) =  uint8(Byte4);
R_Objects_out.StatusFrame(1,5)=   uint8(Byte5);
R_Objects_out.StatusFrame(1,6) =  uint8(Byte6);
R_Objects_out.StatusFrame(1,7) =  uint8(Byte7);
R_Objects_out.StatusFrame(1,8) =  uint8(Byte8);

R_Objects_out.received_frames1 = uint8(0);
R_Objects_out.received_frames2 = uint8(0);
R_Objects_out.isComplete = false;

elseif (R_Objects_in.ObF1_on == true)

R_Objects_out.received_frames1 = R_Objects_in.received_frames1+1;

R_Objects_out.Frames1(1,R_Objects_out.received_frames1) =  uint8(Byte1);
R_Objects_out.Frames1(2,R_Objects_out.received_frames1) =  uint8(Byte2);
R_Objects_out.Frames1(3,R_Objects_out.received_frames1) =  uint8(Byte3);
R_Objects_out.Frames1(4,R_Objects_out.received_frames1) =  uint8(Byte4);
R_Objects_out.Frames1(5,R_Objects_out.received_frames1)=   uint8(Byte5);
R_Objects_out.Frames1(6,R_Objects_out.received_frames1) =  uint8(Byte6);
R_Objects_out.Frames1(7,R_Objects_out.received_frames1) =  uint8(Byte7);
R_Objects_out.Frames1(8,R_Objects_out.received_frames1) =  uint8(Byte8);


elseif (R_Objects_in.ObF2_on == true)

R_Objects_out.received_frames2 = R_Objects_in.received_frames2+1;

R_Objects_out.Frames2(1,R_Objects_out.received_frames2) =  uint8(Byte1);
R_Objects_out.Frames2(2,R_Objects_out.received_frames2) =  uint8(Byte2);
R_Objects_out.Frames2(3,R_Objects_out.received_frames2) =  uint8(Byte3);
R_Objects_out.Frames2(4,R_Objects_out.received_frames2) =  uint8(Byte4);
R_Objects_out.Frames2(5,R_Objects_out.received_frames2)=   uint8(Byte5);
R_Objects_out.Frames2(6,R_Objects_out.received_frames2) =  uint8(Byte6);
R_Objects_out.Frames2(7,R_Objects_out.received_frames2) =  uint8(Byte7);
R_Objects_out.Frames2(8,R_Objects_out.received_frames2) =  uint8(Byte8);

elseif (R_Objects_out.received_frames1 == 40 && R_Objects_out.received_frames2 == 40)
  
    R_Objects_out.isComplete = true;
    

elseif (R_Objects_in.ObS_on == false && R_Objects_in.ObF2_on == false && R_Objects_in.ObF2_on == false)

    R_Objects_out = R_Objects_in;
    
end


end
